simulink model "c4ModeloCompleto"  (R2020b)
settings: Solver=ode45  StartTime=0.0  StopTime=1.2  MaxStep=1e-5  RelTol=1e-4
PreLoadFcn:
  | c4ModeloCompleto_var
values from neighbouring files (symbols this model uses):
  alfa_cu = 3.9e-3    (= 0.0039)    [c4ModeloCompleto_var.m]
  Beq = bm+(bl)/r^2    (= 1.5637748692e-05)    [c4ModeloCompleto_var.m]    (also in polos_y_ceros.m = bm+(bl)/r^2)
  Cts = 0.818    [c4ModeloCompleto_var.m]
  Jeq = Jm+(Jl/r^2)    (= 6.92649215207e-06)    [c4ModeloCompleto_var.m]    (also in polos_y_ceros.m = Jm+(Jl/r^2))
  lambda_m = 0.01546    [c4ModeloCompleto_var.m]
  Ld = 6.6e-3    (= 0.0066)    [c4ModeloCompleto_var.m]
  Lls = 0.8e-3    (= 0.0008)    [c4ModeloCompleto_var.m]
  Lq = 5.8e-3    (= 0.0058)    [c4ModeloCompleto_var.m]
  Pp = 3    [c4ModeloCompleto_var.m]
  r = 314.3008    [c4ModeloCompleto_var.m]
  R_Ref = 1.02    [c4ModeloCompleto_var.m]
  Rts_amb = 146.7    [c4ModeloCompleto_var.m]
  TREF = 40    [c4ModeloCompleto_var.m]
undefined symbols (not defined in the file or in its folder): sigbuilder_block, Tamb
settings Model: Creator=agustin  LastModifiedBy=agustin
settings DataIOCC: ReturnWorkspaceOutputs=off
settings DebuggingCC: ArithmeticOperatorsInVariantConditions=warning
settings SFSimCC: SimUseLocalCustomCode=off  CustomCodeUndefinedFunction=UseInterfaceOnly
settings RTWCC: RTWUseLocalCustomCode=off
settings CodeAppCC: StateflowObjectComments=on

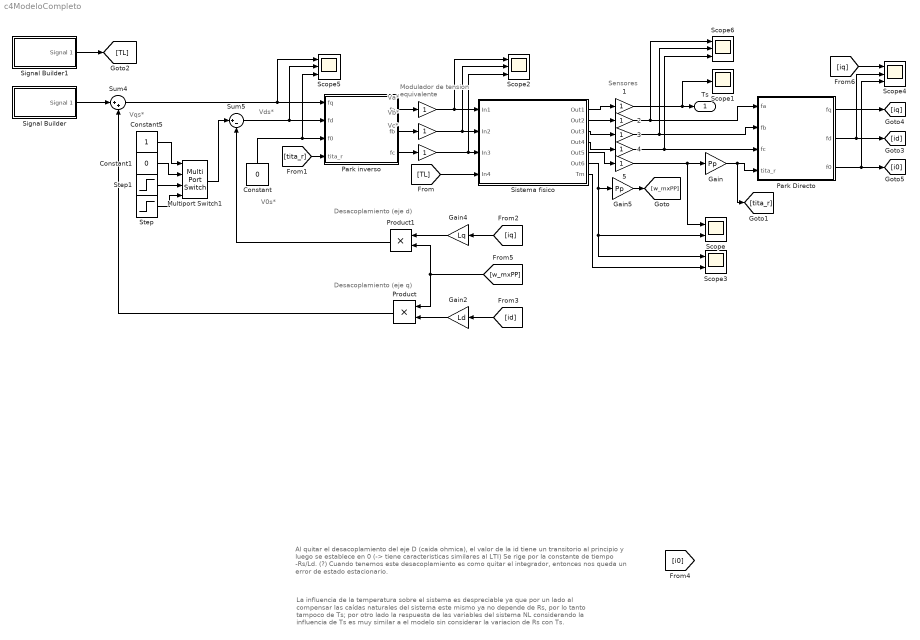
== system c4ModeloCompleto ==
  note: Sensores
  note: La influencia de la temperatura sobre el sistema es despreciable ya que por un lado al compensar las caídas naturales del sistema este mismo ya no depende de Rs, por lo tanto tampoco de Ts; por otro lado la respuesta de las variables del sistema NL considerando la influencia de Ts es muy similar a el modelo sin considerar la variacion de Rs con Ts.
  note: Al quitar el desacoplamiento del eje D (caida ohmica), el valor de la id tiene
      | un transitorio al principio y luego se establece en 0 (-> tiene caracteristicas similares al LTI)
      | Se rige por la constante de tiempo -Rs/Ld.
      | (?) Cuando tenemos este desacoplamiento es como quitar el integrador, entonces nos queda un error de estado
      | estacionario.
  note: V0s*
  note: Vds*
  note: Desacoplamiento (eje d)
  note: Vqs*
  note: Modulador de tension
      | equivalente
  note: Vc*
  note: Vb*
  note: Va*
  note: Desacoplamiento (eje q)
   {,,,1..5} (8 alike) : Gain
  Constant : Constant  Value=0
  Constant1 : Constant  Value=0
  Constant5 : Constant
  Gain : Gain  Gain=Pp
  Gain2 : Gain  Gain=Ld
  Gain4 : Gain  Gain=Lq
  Gain5 : Gain  Gain=Pp
  Multiport Switch1 : MultiPortSwitch
  Park Directo : MATLAB Function  TreatAsAtomicUnit=on
  Park inverso : MATLAB Function  TreatAsAtomicUnit=on
  Product : Product
  Product1 : Product
  Scope : Scope  NumInputPorts=2
  Scope1 : Scope
  Scope{2,4..6} (4 alike) : Scope  NumInputPorts=3
  Scope3 : Scope  NumInputPorts=2
  Signal Builder : Subsystem  Tag=STV Subsys  LoadFcn=sigbuilder_block('load');  StartFcn=sigbuilder_block('start');  StopFcn=sigbuilder_block('stop');  ClipboardFcn=sigbuilder_block('clipboard');  mask(Sigbuilder block){tuvar=[0:10]}
      mask help: Simulink:masks:SigbuilderBlock_MD
      mask init:
      | if ~strcmp(get_param(bdroot(gcbh),'SimulationStatus'),'stopped') tuvar = sigbuilder_block('maskInit'); end
      settings: CopyFcn=sigbuilder_block('copy');  DeleteFcn=sigbuilder_block('delete');  ModelCloseFcn=sigbuilder_block('modelClose');  PreSaveFcn=sigbuilder_block('preSave');  PauseFcn=sigbuilder_block('pause');  ContinueFcn=sigbuilder_block('continue');  NameChangeFcn=sigbuilder_block('namechange');  OpenFcn=sigbuilder_block('open',[437.25 154.5 550.5 357 ]);  CloseFcn=sigbuilder_block('close');
      mask Display: plot(0, 0, 100, 100,[2, 2, 32, 32, 2], [68, 8, 8, 68, 68],[32, 2], [38, 38], [32, 19, 2],[53, 60, 44], [32, 17, 17, 2],[16, 16, 31, 31]);txt = getActiveGroup(gcbh);text(2, 100, txt,'verticalAlignment', 'top');
  Signal Builder1 : Subsystem  Tag=STV Subsys  LoadFcn=sigbuilder_block('load');  StartFcn=sigbuilder_block('start');  StopFcn=sigbuilder_block('stop');  ClipboardFcn=sigbuilder_block('clipboard');  mask(Sigbuilder block){tuvar=[0:10]}
      mask help: Simulink:masks:SigbuilderBlock_MD
      mask init:
      | if ~strcmp(get_param(bdroot(gcbh),'SimulationStatus'),'stopped') tuvar = sigbuilder_block('maskInit'); end
      settings: CopyFcn=sigbuilder_block('copy');  DeleteFcn=sigbuilder_block('delete');  ModelCloseFcn=sigbuilder_block('modelClose');  PreSaveFcn=sigbuilder_block('preSave');  PauseFcn=sigbuilder_block('pause');  ContinueFcn=sigbuilder_block('continue');  NameChangeFcn=sigbuilder_block('namechange');  OpenFcn=sigbuilder_block('open',[0 0 1024.5 511.5 ]);  CloseFcn=sigbuilder_block('close');
      mask Display: plot(0, 0, 100, 100,[2, 2, 32, 32, 2], [68, 8, 8, 68, 68],[32, 2], [38, 38], [32, 19, 2],[53, 60, 44], [32, 17, 17, 2],[16, 16, 31, 31]);txt = getActiveGroup(gcbh);text(2, 100, txt,'verticalAlignment', 'top');
  Sistema fisico : Subsystem
  Step : Step  Time=0.5  After=-1.9596  SampleTime=0
  Step1 : Step  Time=0.5  After=1.9596  SampleTime=0
  Sum4 : Sum  Inputs=|++
  Sum5 : Sum  Inputs=|+-
  Ts : Outport  VectorParamsAs1DForOutWhenUnconnected=off
  wires:
  Park inverso/1(fa) -> " "/1
  Park inverso/2(fb) -> " "/1
  Park inverso/3(fc) -> " "/1
  Product/1 -> Sum4/2
  Gain4/1 -> Product1/1
  Product1/1 -> Sum5/2
  " 1"/1 -> Scope1/1, Ts/1
  [iq] -> Gain4/1
  Sum5/1 -> Park inverso/2(fd), Scope5/2
  Gain2/1 -> Product/2
  Constant/1 -> Park inverso/3(f0), Scope5/3
  [id] -> Gain2/1
  Park Directo/2(fd) -> Scope4/2, [id]
  Park Directo/1(fq) -> [iq]
  Sum4/1 -> Park inverso/1(fq), Scope5/1
  [w_mxPP] -> Product1/2, Product/1
  " "/1 -> Sistema fisico/1(In1), Scope2/1
  " "/1 -> Scope2/3, Sistema fisico/3(In3)
  Sistema fisico/1(Out1) -> " 1"/1
  Sistema fisico/2(Out2) -> " 2"/1
  Sistema fisico/3(Out3) -> " 3"/1
  Sistema fisico/4(Out4) -> " 4"/1
  [TL] -> Sistema fisico/4(In4)
  Gain5/1 -> [w_mxPP]
  Park Directo/3(f0) -> Scope4/3, [i0]
  [iq] -> Scope4/1
  Signal Builder/1(Signal 1) -> Sum4/1
  Signal Builder1/1(Signal 1) -> [TL]
  Sistema fisico/6(Out6) -> Gain5/1, Scope3/1, Scope/2
  Multiport Switch1/1 -> Sum5/1
  " "/1 -> Sistema fisico/2(In2), Scope2/2
  " 3"/1 -> Scope6/2, Park Directo/2(fb)
  " 4"/1 -> Scope6/3, Park Directo/3(fc)
  " 2"/1 -> Scope6/1, Park Directo/1(fa)
  Sistema fisico/7(Tm) -> Scope3/2
  " 5"/1 -> Gain/1, Scope/1
  Sistema fisico/5(Out5) -> " 5"/1
  Gain/1 -> [tita_r], Park Directo/4(tita_r)
  [tita_r] -> Park inverso/4(tita_r)
  Constant1/1 -> Multiport Switch1/2
  Constant5/1 -> Multiport Switch1/1
  Step/1 -> Multiport Switch1/4
  Step1/1 -> Multiport Switch1/3

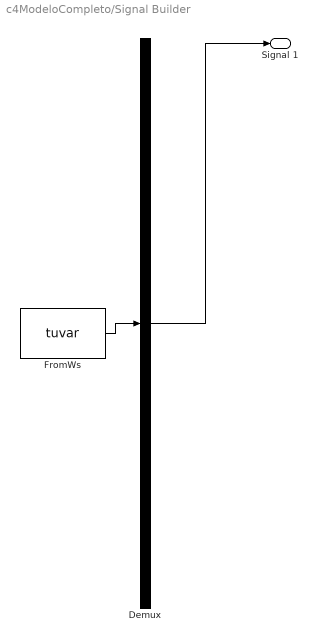
== system c4ModeloCompleto/Signal Builder ==
  Demux : Demux  Tag=STV Demux  Outputs=1
      settings: DisplayOption=none
  FromWs : FromWorkspace  Tag=STV FromWs  VariableName=tuvar
      SigBuilderData=|
      | common.afterFinalStr = 'Extrapolate'
      | common.sampleTime = 0
      | dataSet.timeRange = [0 10]
      | dataSet.name = 'Group 1'
      | sbobj.Groups.Name = 'Group 1'
      | sbobj.Groups.Signals.Name = 'Signal 1'
      | sbobj.Groups.Signals.XData = [0 0.1 0.1 0.7 0.7 10]
      | sbobj.Groups.Signals.YData = [0 0 19.596 19.596 0 0]
  Signal 1 : Outport  Tag=STV Outport  VectorParamsAs1DForOutWhenUnconnected=off
  wires:
  Demux/1 -> Signal 1/1
  FromWs/1 -> Demux/1

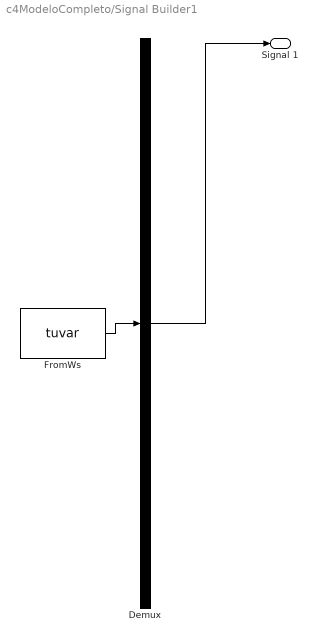
== system c4ModeloCompleto/Signal Builder1 ==
  Demux : Demux  Tag=STV Demux  Outputs=1
      settings: DisplayOption=none
  FromWs : FromWorkspace  Tag=STV FromWs  VariableName=tuvar
      SigBuilderData=|
      | common.afterFinalStr = 'Extrapolate'
      | common.sampleTime = 0
      | dataSet.timeRange = [0 10]
      | dataSet.name = 'Group 1'
      | sbobj.Groups.Name = 'Group 1'
      | sbobj.Groups.Signals.Name = 'Signal 1'
      | sbobj.Groups.Signals.XData = [0 0.3 0.3 0.5 0.5 0.9 0.9 10]
      | sbobj.Groups.Signals.YData = [0 0 6.28 6.28 -6.28 -6.28 0 0]
  Signal 1 : Outport  Tag=STV Outport  VectorParamsAs1DForOutWhenUnconnected=off
  wires:
  Demux/1 -> Signal 1/1
  FromWs/1 -> Demux/1

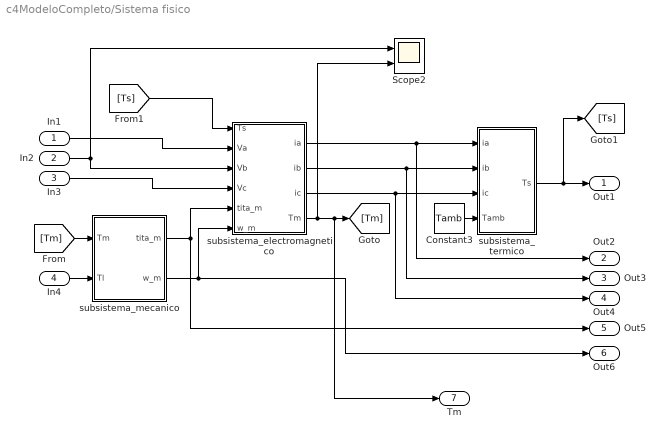
== system c4ModeloCompleto/Sistema fisico ==
  In1 : Inport
  In2 : Inport  Port=2
  In3 : Inport  Port=3
  In4 : Inport  Port=4
  Constant3 : Constant  Value=Tamb
  Scope2 : Scope  NumInputPorts=2
  "subsistema_electromagnetico " : Subsystem
  "subsistema_mecanico " : Subsystem
  subsistema_termico : Subsystem
  Out1 : Outport  VectorParamsAs1DForOutWhenUnconnected=off
  Out2 : Outport  Port=2  VectorParamsAs1DForOutWhenUnconnected=off
  Out3 : Outport  Port=3  VectorParamsAs1DForOutWhenUnconnected=off
  Out4 : Outport  Port=4  VectorParamsAs1DForOutWhenUnconnected=off
  Out5 : Outport  Port=5  VectorParamsAs1DForOutWhenUnconnected=off
  Out6 : Outport  Port=6  VectorParamsAs1DForOutWhenUnconnected=off
  Tm : Outport  Port=7  VectorParamsAs1DForOutWhenUnconnected=off
  wires:
  "subsistema_mecanico "/2(w_m) -> Out6/1, "subsistema_electromagnetico "/6(w_m)
  "subsistema_electromagnetico "/3(ic) -> Out4/1, subsistema_termico/3("ic ")
  In2/1 -> "subsistema_electromagnetico "/3(Vb), Scope2/1
  [Tm] -> "subsistema_mecanico "/1(Tm)
  In4/1 -> "subsistema_mecanico "/2(Tl)
  "subsistema_electromagnetico "/1(ia) -> Out2/1, subsistema_termico/1(ia)
  "subsistema_electromagnetico "/4(Tm) -> Scope2/2, Tm/1, [Tm]
  In1/1 -> "subsistema_electromagnetico "/2(Va)
  Constant3/1 -> subsistema_termico/4(Tamb)
  "subsistema_electromagnetico "/2(ib) -> Out3/1, subsistema_termico/2(ib)
  In3/1 -> "subsistema_electromagnetico "/4(Vc)
  "subsistema_mecanico "/1("tita_m ") -> Out5/1, "subsistema_electromagnetico "/5(tita_m)
  subsistema_termico/1(Ts) -> [Ts], Out1/1
  [Ts] -> "subsistema_electromagnetico "/1(Ts)

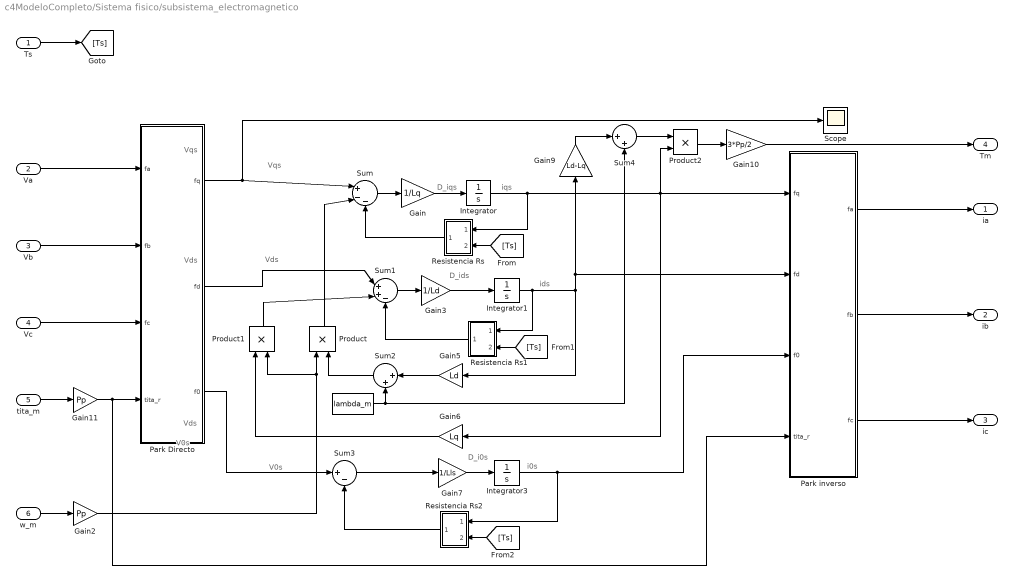
== system c4ModeloCompleto/Sistema fisico/subsistema_electromagnetico  ==
  note: V0s
  note: Vds
  note: Vqs
  note: Vds
  note: Vqs
  note: V0s
  note: Vds
  note: i0s
  note: D_i0s
  note: D_ids
  note: ids
  note: iqs
  note: D_iqs
  Ts : Inport
  Va : Inport  Port=2
  Vb : Inport  Port=3
  Vc : Inport  Port=4
  tita_m : Inport  Port=5
  w_m : Inport  Port=6
  " " : Constant  Value=lambda_m
  Gain : Gain  Gain=1/Lq
  Gain10 : Gain  Gain=3*Pp/2
  Gain11 : Gain  Gain=Pp
  Gain2 : Gain  Gain=Pp
  Gain3 : Gain  Gain=1/Ld
  Gain5 : Gain  Gain=Ld
  Gain6 : Gain  Gain=Lq
  Gain7 : Gain  Gain=1/Lls
  Gain9 : Gain  Gain=Ld-Lq
  Integrator : Integrator
  Integrator1 : Integrator
  Integrator3 : Integrator
  Park Directo : MATLAB Function  TreatAsAtomicUnit=on
  Park inverso : MATLAB Function  TreatAsAtomicUnit=on
  Product : Product
  Product1 : Product
  Product2 : Product
  Resistencia Rs : Subsystem
  Resistencia Rs1 : Subsystem
  Resistencia Rs2 : Subsystem
  Scope : Scope
  Sum : Sum  Inputs=|+--
  Sum1 : Sum  Inputs=|++-
  Sum2 : Sum  Inputs=|++
  Sum3 : Sum  Inputs=|+-
  Sum4 : Sum  Inputs=|++
  ia : Outport  VectorParamsAs1DForOutWhenUnconnected=off
  ib : Outport  Port=2  VectorParamsAs1DForOutWhenUnconnected=off
  ic : Outport  Port=3  VectorParamsAs1DForOutWhenUnconnected=off
  Tm : Outport  Port=4  VectorParamsAs1DForOutWhenUnconnected=off
  wires:
  Product/1 -> Sum/2
  w_m/1 -> Gain2/1
  Product1/1 -> Sum1/2
  Gain2/1 -> Product1/2, Product/1
  Park Directo/3(f0) -> Sum3/1
  Integrator/1 -> Resistencia Rs/1(In1), Product2/2, Park inverso/1(fq), Gain6/1
  Sum2/1 -> Product/2
  Sum3/1 -> Gain7/1
  Park Directo/1(fq) -> Scope/1, Sum/1
  Sum/1 -> Gain/1
  Gain3/1 -> Integrator1/1
  Park Directo/2(fd) -> Sum1/1
  Sum1/1 -> Gain3/1
  Gain5/1 -> Sum2/1
  Gain/1 -> Integrator/1
  Gain6/1 -> Product1/1
  Resistencia Rs/1(In*Rs) -> Sum/3
  " "/1 -> Sum4/2, Sum2/2
  Gain7/1 -> Integrator3/1
  Gain9/1 -> Sum4/1
  Sum4/1 -> Product2/1
  Product2/1 -> Gain10/1
  Gain10/1 -> Tm/1
  Vb/1 -> Park Directo/2(fb)
  Va/1 -> Park Directo/1(fa)
  Vc/1 -> Park Directo/3(fc)
  tita_m/1 -> Gain11/1
  Gain11/1 -> Park inverso/4(tita_r), Park Directo/4(tita_r)
  Park inverso/1(fa) -> ia/1
  Park inverso/2(fb) -> ib/1
  Park inverso/3(fc) -> ic/1
  Ts/1 -> [Ts]
  [Ts] -> Resistencia Rs/2(Ts)
  Resistencia Rs1/1(In*Rs) -> Sum1/3
  Integrator1/1 -> Gain9/1, Park inverso/2(fd), Gain5/1, Resistencia Rs1/1(In1)
  [Ts] -> Resistencia Rs1/2(Ts)
  Resistencia Rs2/1(In*Rs) -> Sum3/2
  Integrator3/1 -> Resistencia Rs2/1(In1), Park inverso/3(f0)
  [Ts] -> Resistencia Rs2/2(Ts)

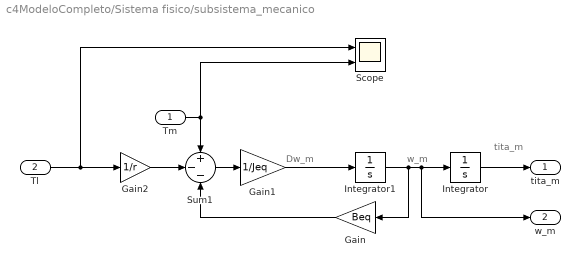
== system c4ModeloCompleto/Sistema fisico/subsistema_mecanico  ==
  note: Dw_m
  note: w_m
  note: tita_m
  Tm : Inport
  Tl : Inport  Port=2
  Gain : Gain  Gain=Beq
  Gain1 : Gain  Gain=1/Jeq
  Gain2 : Gain  Gain=1/r
  Integrator : Integrator
  Integrator1 : Integrator
  Scope : Scope  NumInputPorts=2
  Sum1 : Sum  Inputs=+--
  "tita_m " : Outport  VectorParamsAs1DForOutWhenUnconnected=off
  w_m : Outport  Port=2  VectorParamsAs1DForOutWhenUnconnected=off
  wires:
  Gain1/1 -> Integrator1/1
  Integrator1/1 -> Integrator/1, w_m/1, Gain/1
  Integrator/1 -> "tita_m "/1
  Sum1/1 -> Gain1/1
  Tm/1 -> Sum1/1, Scope/2
  Gain/1 -> Sum1/3
  Gain2/1 -> Sum1/2
  Tl/1 -> Scope/1, Gain2/1

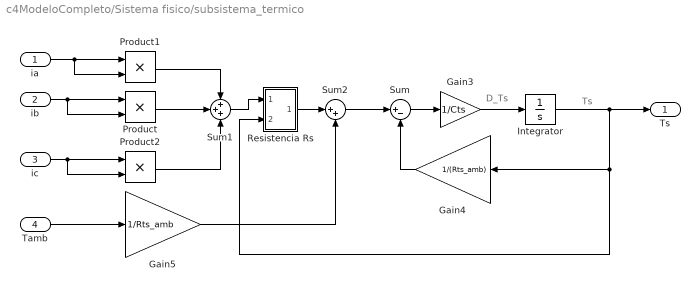
== system c4ModeloCompleto/Sistema fisico/subsistema_termico ==
  note: Ts
  note: D_Ts
  ia : Inport
  ib : Inport  Port=2
  "ic " : Inport  Port=3
  Tamb : Inport  Port=4
  Gain3 : Gain  Gain=1/Cts
  Gain4 : Gain  Gain=1/(Rts_amb)
  Gain5 : Gain  Gain=1/Rts_amb
  Integrator : Integrator  InitialCondition=40
  Product : Product
  Product1 : Product
  Product2 : Product
  Resistencia Rs : Subsystem
  Sum : Sum  Inputs=|+-
  Sum1 : Sum  Inputs=+++
  Sum2 : Sum  Inputs=|++
  Ts : Outport  VectorParamsAs1DForOutWhenUnconnected=off
  wires:
  Gain4/1 -> Sum/2
  Sum1/1 -> Resistencia Rs/1(In1)
  Product2/1 -> Sum1/3
  Product/1 -> Sum1/2
  Integrator/1 -> Ts/1, Resistencia Rs/2(Ts), Gain4/1
  ib/1 -> Product/2, Product/1
  "ic "/1 -> Product2/2, Product2/1
  Sum2/1 -> Sum/1
  Product1/1 -> Sum1/1
  Gain5/1 -> Sum2/2
  Resistencia Rs/1(In*Rs) -> Sum2/1
  ia/1 -> Product1/2, Product1/1
  Tamb/1 -> Gain5/1
  Gain3/1 -> Integrator/1
  Sum/1 -> Gain3/1

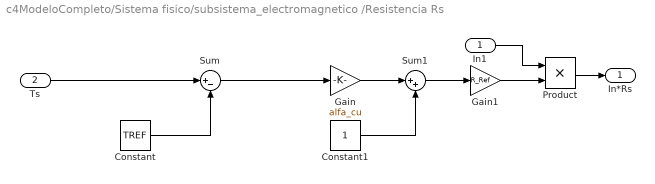
== system c4ModeloCompleto/Sistema fisico/subsistema_electromagnetico /Resistencia Rs ==
  In1 : Inport
  Ts : Inport  Port=2
  Constant : Constant  Value=TREF
  Constant1 : Constant
  Gain : Gain  Gain=alfa_cu
  Gain1 : Gain  Gain=R_Ref
  Product : Product
  Sum : Sum  Inputs=|+-
  Sum1 : Sum  Inputs=|++
  In*Rs : Outport
  wires:
  Constant/1 -> Sum/2
  Gain/1 -> Sum1/1
  Gain1/1 -> Product/2
  Sum1/1 -> Gain1/1
  Sum/1 -> Gain/1
  Ts/1 -> Sum/1
  Constant1/1 -> Sum1/2
  In1/1 -> Product/1
  Product/1 -> In*Rs/1

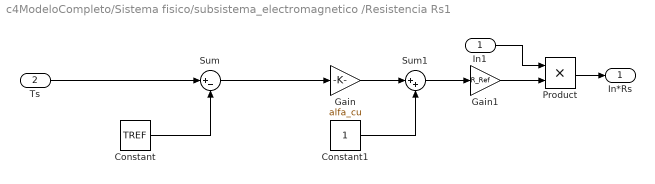
== system c4ModeloCompleto/Sistema fisico/subsistema_electromagnetico /Resistencia Rs1 ==
  In1 : Inport
  Ts : Inport  Port=2
  Constant : Constant  Value=TREF
  Constant1 : Constant
  Gain : Gain  Gain=alfa_cu
  Gain1 : Gain  Gain=R_Ref
  Product : Product
  Sum : Sum  Inputs=|+-
  Sum1 : Sum  Inputs=|++
  In*Rs : Outport
  wires:
  Constant/1 -> Sum/2
  Gain/1 -> Sum1/1
  Gain1/1 -> Product/2
  Sum1/1 -> Gain1/1
  Sum/1 -> Gain/1
  Ts/1 -> Sum/1
  Constant1/1 -> Sum1/2
  In1/1 -> Product/1
  Product/1 -> In*Rs/1

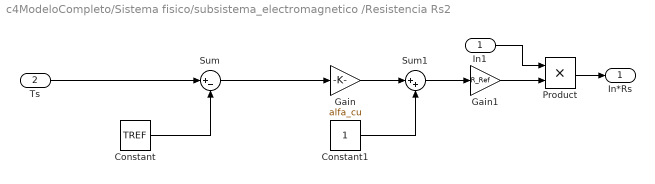
== system c4ModeloCompleto/Sistema fisico/subsistema_electromagnetico /Resistencia Rs2 ==
  In1 : Inport
  Ts : Inport  Port=2
  Constant : Constant  Value=TREF
  Constant1 : Constant
  Gain : Gain  Gain=alfa_cu
  Gain1 : Gain  Gain=R_Ref
  Product : Product
  Sum : Sum  Inputs=|+-
  Sum1 : Sum  Inputs=|++
  In*Rs : Outport
  wires:
  Constant/1 -> Sum/2
  Gain/1 -> Sum1/1
  Gain1/1 -> Product/2
  Sum1/1 -> Gain1/1
  Sum/1 -> Gain/1
  Ts/1 -> Sum/1
  Constant1/1 -> Sum1/2
  In1/1 -> Product/1
  Product/1 -> In*Rs/1

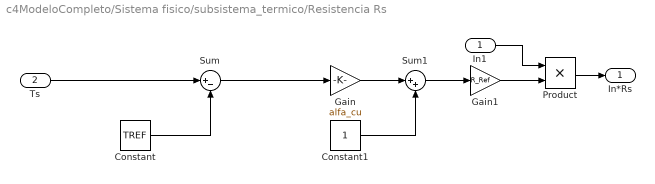
== system c4ModeloCompleto/Sistema fisico/subsistema_termico/Resistencia Rs ==
  In1 : Inport
  Ts : Inport  Port=2
  Constant : Constant  Value=TREF
  Constant1 : Constant
  Gain : Gain  Gain=alfa_cu
  Gain1 : Gain  Gain=R_Ref
  Product : Product
  Sum : Sum  Inputs=|+-
  Sum1 : Sum  Inputs=|++
  In*Rs : Outport
  wires:
  Constant/1 -> Sum/2
  Gain/1 -> Sum1/1
  Gain1/1 -> Product/2
  Sum1/1 -> Gain1/1
  Sum/1 -> Gain/1
  Ts/1 -> Sum/1
  Constant1/1 -> Sum1/2
  In1/1 -> Product/1
  Product/1 -> In*Rs/1

== matlab function c4ModeloCompleto/Park inverso ==
  data: fq input; fd input; f0 input; tita_r input; fa output; fb output; fc output
function [fa, fb, fc] = t_park_inv(fq, fd , f0, tita_r)


park_MATRIZ = [cos(tita_r)        sin(tita_r)        1; 
               cos(tita_r-2*pi/3) sin(tita_r-2*pi/3) 1;
               cos(tita_r+2*pi/3) sin(tita_r+2*pi/3) 1];
                 
park_inv = park_MATRIZ * [fq;fd;f0];
fa = park_inv(1);
fb = park_inv(2);
fc = park_inv(3);
end

== matlab function c4ModeloCompleto/Sistema fisico/subsistema_electromagnetico /Park Directo ==
  data: fa input; fq output; fb input; fc input; tita_r input; fd output; f0 output
function [fq,fd,f0]     = t_park(fa,fb,fc,tita_r)

park_MATRIZ = [cos(tita_r) cos(tita_r-2*pi/3) cos(tita_r+2*pi/3); 
               sin(tita_r) sin(tita_r-2*pi/3) sin(tita_r+2*pi/3);
                  0.5           0.5            0.5];
                 
park_dir = (2/3) * park_MATRIZ * [fa;fb;fc];
fq = park_dir(1);
fd = park_dir(2);
f0 = park_dir(3);

end

== matlab function c4ModeloCompleto/Sistema fisico/subsistema_electromagnetico /Park inverso ==
  data: fq input; fd input; f0 input; tita_r input; fa output; fb output; fc output
function [fa, fb, fc] = t_park_inv(fq, fd , f0, tita_r)


park_MATRIZ = [cos(tita_r)        sin(tita_r)        1; 
               cos(tita_r-2*pi/3) sin(tita_r-2*pi/3) 1;
               cos(tita_r+2*pi/3) sin(tita_r+2*pi/3) 1];
                 
park_inv = park_MATRIZ * [fq;fd;f0];
fa = park_inv(1);
fb = park_inv(2);
fc = park_inv(3);
end

== matlab function c4ModeloCompleto/Park Directo ==
  data: fa input; fq output; fb input; fc input; tita_r input; fd output; f0 output
function [fq,fd,f0]     = t_park(fa,fb,fc,tita_r)

park_MATRIZ = [cos(tita_r) cos(tita_r-2*pi/3) cos(tita_r+2*pi/3); 
               sin(tita_r) sin(tita_r-2*pi/3) sin(tita_r+2*pi/3);
                  0.5           0.5            0.5];
                 
park_dir = (2/3) * park_MATRIZ * [fa;fb;fc];
fq = park_dir(1);
fd = park_dir(2);
f0 = park_dir(3);
end
